simulink model "project"  (R2025a)
settings: Solver=VariableStepAuto  StartTime=0.0  StopTime=20  RelTol=1e-3
undefined symbols (not defined in the file or in its folder): p
settings Model: Creator=rgarc  LastModifiedBy=rgarc

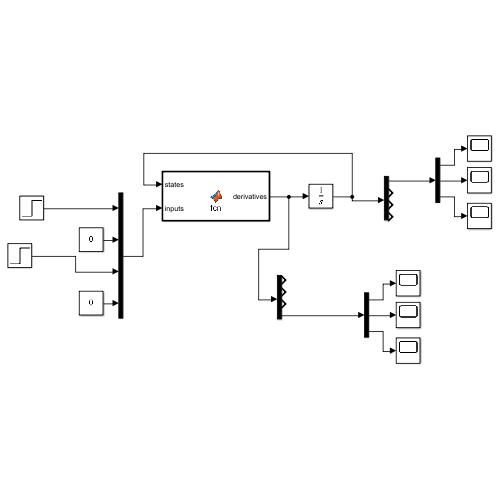
[thumbnail: Simulink's stored preview of the top-level diagram]
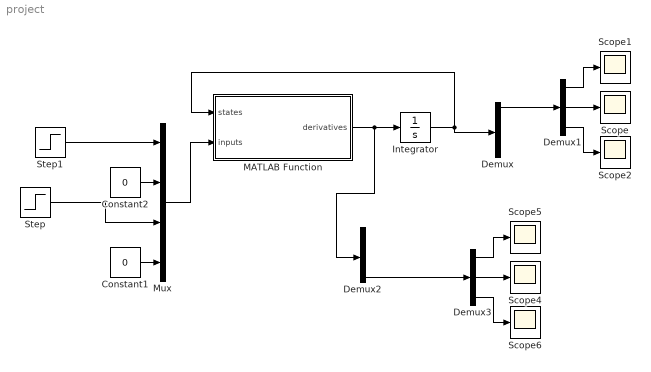
== system project ==
  Constant1 : Constant  Value=0
  Constant2 : Constant  Value=0
  Demux : Demux
  Demux1 : Demux  Outputs=3
  Demux2 : Demux
  Demux3 : Demux  Outputs=3
  Integrator : Integrator
  MATLAB Function : MATLAB Function  TreatAsAtomicUnit=on
  Mux : Mux
  Scope{,1..2,4..6} (6 alike) : Scope
      Scope settings: ActiveDisplayYMinimum=-1  ActiveDisplayYMaximum=1
      Scope1 settings: ActiveDisplayYMinimum=-0.72892081300229672  ActiveDisplayYMaximum=1.2797034818614446
      Scope2 settings: ActiveDisplayYMinimum=-1  ActiveDisplayYMaximum=1  DataLoggingVariableName=ScopeData2
      Scope4 settings: ActiveDisplayYMinimum=-1  ActiveDisplayYMaximum=1  DataLoggingVariableName=ScopeData4
      Scope5 settings: ActiveDisplayYMinimum=-1  ActiveDisplayYMaximum=1  DataLoggingVariableName=ScopeData5
      Scope6 settings: ActiveDisplayYMinimum=-1  ActiveDisplayYMaximum=1  DataLoggingVariableName=ScopeData6
  Step : Step  Time=10  After=10  SampleTime=0
  Step1 : Step  Time=0  After=p.g*p.m  SampleTime=0
  wires:
  Integrator/1 -> Demux/1, MATLAB Function/1(states)
  Mux/1 -> MATLAB Function/2(inputs)
  Step1/1 -> Mux/1
  Constant1/1 -> Mux/4
  Constant2/1 -> Mux/2
  Step/1 -> Mux/3
  Demux1/3 -> Scope2/1
  Demux1/1 -> Scope1/1
  Demux/1 -> Demux1/1
  Demux1/2 -> Scope/1
  MATLAB Function/1(derivatives) -> Demux2/1, Integrator/1
  Demux3/1 -> Scope5/1
  Demux2/4 -> Demux3/1
  Demux3/2 -> Scope4/1
  Demux3/3 -> Scope6/1

== matlab function project/MATLAB Function ==
  data: states input size=12; derivatives output size=12; inputs input size=4; p parameter
function derivatives = fcn(states, inputs, p)

xidot  = states(4:6);
eta    = states(7:9); 
etadot = states(10:12);

phi = eta(1);
theta = eta(2);
psi = eta(3);

phid = etadot(1);
thetad = etadot(2);

W = [1,0,-sin(theta);0, cos(phi), sin(phi)*cos(theta); 0, -sin(phi), cos(phi)*cos(theta)];
dotW = [0,0,-thetad*cos(theta);0, phid*-sin(phi), phid*cos(phi)*cos(theta) - thetad* sin(phi)*sin(theta); 0, -phid*cos(phi), -phid*sin(phi)*cos(theta) - thetad*cos(phi)*sin(theta)];

R_x = [1,0,0;0,cos(phi), -sin(phi); 0,sin(phi), cos(phi)];
R_y = [cos(theta), 0, sin(theta); 0, 1, 0; -sin(theta),0,cos(theta)];
R_z = [cos(psi), -sin(psi), 0; sin(psi), cos(psi), 0; 0,0,1];

R_euler = R_z * R_y * R_x;
I_body = [p.Ixx, 0,0;0,p.Iyy, 0; 0,0,p.Izz];

friction_force = -p.kD * xidot;

thrust = inputs(1);
torque = inputs(2:4);

weta_cross_iweta = cross((W * eta), (I_body * W * eta));

etadotdot = W \ (I_body \ (torque - weta_cross_iweta - dotW * etadot));

xidotdot = R_euler * [0;0;thrust/p.m] + friction_force - [0;0;p.g];

% Xdot = xidot(1);
% Xdotdot = thrust/p.m * (sin(psi) * sin(phi) + cos(psi) * sin(theta) * cos(phi)) - p.kD / p.m  * Xdot;
% Ydot = xidot(2);
% Ydotdot = thrust/p.m * (sin(psi) * sin(theta) * cos(phi) - cos(psi) * sin(phi)) - p.kD / p.m  * Ydot;
% Zdot = xidot(3);
% Zdotdot = -p.g + 1/p.m * (cos(theta) * cos(phi)) * thrust - p.kD / p.m * Zdot;

% xidotdot = [Xdotdot;Ydotdot;Zdotdot];


derivatives = [xidot;xidotdot;etadot;etadotdot];
